simulink model "ACtoDC_WPT_current_DC"  (R2018a)
settings: Solver=FixedStepAuto  StartTime=0.0  StopTime=stopTime  FixedStep=sampleTime  RelTol=1e-3
InitFcn:
  | fs=150e3; %Hz
  | wo=2*pi*fs;
  | stopTime=0.1;
  | sampleTime=1e-8;
  | Lp=81e-6;
  | Ls=66e-6;
  | Cs=1/ (Ls*4*pi*pi*150e3*150e3);
  | Cp=1/ (Lp*4*pi*pi*150e3*150e3);
  | RLOAD=20
  | k=0.2;
  | M=sqrt(Lp*Ls)*k;
  | Cout=1e-6; %F
  | fs=150e3*sqrt(1+k^2); %Hz
values from neighbouring files (symbols this model uses):
  Rp = 0.3    [Calculation.m]
libraries: powerlib x37
settings Model: Creator=enes_  LastModifiedBy=enes_

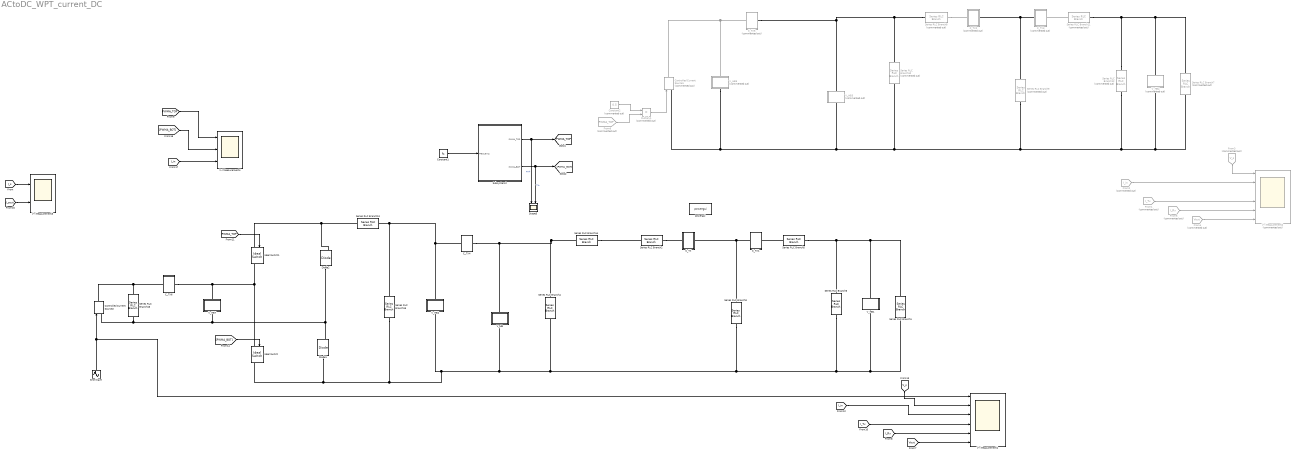
== system ACtoDC_WPT_current_DC ==
  C_TX : Subsystem
  C_TX1 : Subsystem
  C_TX2 : Subsystem  Commented=on
  C_TX3 : Subsystem  Commented=on
  C_TX4 : Subsystem
  C_TX5 : Subsystem  Commented=on
  C_TX6 : Subsystem
  Constant1 : Constant  Value=fs
  Constant2 : Constant  Commented=on  Value=0.5
  Controlled Current Source1 : powerlib/Electrical Sources/Controlled Current Source  Commented=on  Initialize=on  Source_Type=AC  Amplitude=0  Phase=0  Frequency=0  Measurements=None
  Controlled Current Source2 : powerlib/Electrical Sources/Controlled Current Source  Initialize=on  Source_Type=AC  Amplitude=0  Phase=0  Frequency=0  Measurements=None
  Diode1 : powerlib/Power Electronics/Diode  Ron=0.01  Lon=0  Vf=0.8  IC=0  UseSnubber=0  Rs=500  Cs=250e-9  Measurements=on
  Diode2 : powerlib/Power Electronics/Diode  Ron=0.01  Lon=0  Vf=0.8  IC=0  UseSnubber=0  Rs=500  Cs=250e-9  Measurements=on
  From1 : From  Commented=on  GotoTag=I_Tx  TagVisibility=global
  From2 : From  Commented=on  GotoTag=I_in  TagVisibility=global
  From3 : From  Commented=on  GotoTag=V_s  TagVisibility=global
  From4 : From  Commented=on  GotoTag=Vout  TagVisibility=global
  From5 : From  Commented=on  GotoTag=I_Rx  TagVisibility=global
  From6 : From  Commented=on  GotoTag=PWMA_TOP  TagVisibility=global
  Ideal Switch : powerlib/Power Electronics/Ideal Switch  Ron=0.01  Lon=0  IC=0  Rs=1e5  Cs=inf  Measurements=on
  Ideal Switch1 : powerlib/Power Electronics/Ideal Switch  Ron=0.01  Lon=0  IC=0  Rs=1e5  Cs=inf  Measurements=on
  Multiply1 : Product  Commented=on
  Scope3 : Scope  NumInputPorts=2
  Series RLC Branch1 : powerlib/Elements/Series RLC Branch  LConnTagsString=__new0  RConnTagsString=__new0  BranchType=R  Resistance=RLOAD*10  Inductance=Lp  SetiL0=off  InitialCurrent=0  Capacitance=Cp  Setx0=off  InitialVoltage=0  Measurements=None
  Series RLC Branch10 : powerlib/Elements/Series RLC Branch  Commented=on  LConnTagsString=__new0  RConnTagsString=__new0  BranchType=C  Resistance=Rp  Inductance=Lp  SetiL0=off  InitialCurrent=0  Capacitance=Cp  Setx0=off  InitialVoltage=0  Measurements=None
  Series RLC Branch11 : powerlib/Elements/Series RLC Branch  Commented=on  LConnTagsString=__new0  RConnTagsString=__new0  BranchType=L  Resistance=Rp  Inductance=Ls-M  SetiL0=off  InitialCurrent=0  Capacitance=Cp  Setx0=off  InitialVoltage=0  Measurements=None
  Series RLC Branch12 : powerlib/Elements/Series RLC Branch  Commented=on  LConnTagsString=__new0  RConnTagsString=__new0  BranchType=C  Resistance=Rp  Inductance=Lp  SetiL0=off  InitialCurrent=0  Capacitance=Cs  Setx0=off  InitialVoltage=0  Measurements=None
  Series RLC Branch13 : powerlib/Elements/Series RLC Branch  LConnTagsString=__new0  RConnTagsString=__new0  BranchType=R  Resistance=Rp  Inductance=Lp  SetiL0=off  InitialCurrent=0  Capacitance=0.01  Setx0=off  InitialVoltage=0  Measurements=None
  Series RLC Branch14 : powerlib/Elements/Series RLC Branch  LConnTagsString=__new0  RConnTagsString=__new0  BranchType=C  Resistance=Rp  Inductance=Lp  SetiL0=off  InitialCurrent=0  Capacitance=Cp*5  Setx0=off  InitialVoltage=0  Measurements=None
  Series RLC Branch15 : powerlib/Elements/Series RLC Branch  LConnTagsString=__new0  RConnTagsString=__new0  BranchType=R  Resistance=10e3  Inductance=Lp  SetiL0=off  InitialCurrent=0  Capacitance=0.01  Setx0=off  InitialVoltage=0  Measurements=None
  Series RLC Branch16 : powerlib/Elements/Series RLC Branch  LConnTagsString=__new0  RConnTagsString=__new0  BranchType=R  Resistance=10e3  Inductance=Lp  SetiL0=off  InitialCurrent=0  Capacitance=0.01  Setx0=off  InitialVoltage=0  Measurements=None
  Series RLC Branch2 : powerlib/Elements/Series RLC Branch  LConnTagsString=__new0  RConnTagsString=__new0  BranchType=L  Resistance=Rp  Inductance=Lp-M  SetiL0=off  InitialCurrent=0  Capacitance=Cp  Setx0=off  InitialVoltage=0  Measurements=None
  Series RLC Branch3 : powerlib/Elements/Series RLC Branch  LConnTagsString=__new0  RConnTagsString=__new0  BranchType=L  Resistance=Rp  Inductance=M  SetiL0=off  InitialCurrent=0  Capacitance=Cp  Setx0=off  InitialVoltage=0  Measurements=None
  Series RLC Branch4 : powerlib/Elements/Series RLC Branch  LConnTagsString=__new0  RConnTagsString=__new0  BranchType=C  Resistance=Rp  Inductance=Lp  SetiL0=off  InitialCurrent=0  Capacitance=Cp/5  Setx0=off  InitialVoltage=0  Measurements=None
  Series RLC Branch5 : powerlib/Elements/Series RLC Branch  LConnTagsString=__new0  RConnTagsString=__new0  BranchType=L  Resistance=Rp  Inductance=Ls-M  SetiL0=off  InitialCurrent=0  Capacitance=Cp  Setx0=off  InitialVoltage=0  Measurements=None
  Series RLC Branch6 : powerlib/Elements/Series RLC Branch  LConnTagsString=__new0  RConnTagsString=__new0  BranchType=C  Resistance=Rp  Inductance=Lp  SetiL0=off  InitialCurrent=0  Capacitance=Cs  Setx0=off  InitialVoltage=0  Measurements=None
  Series RLC Branch7 : powerlib/Elements/Series RLC Branch  Commented=on  LConnTagsString=__new0  RConnTagsString=__new0  BranchType=R  Resistance=RLOAD*10  Inductance=Lp  SetiL0=off  InitialCurrent=0  Capacitance=Cp  Setx0=off  InitialVoltage=0  Measurements=None
  Series RLC Branch8 : powerlib/Elements/Series RLC Branch  Commented=on  LConnTagsString=__new0  RConnTagsString=__new0  BranchType=L  Resistance=Rp  Inductance=Lp-M  SetiL0=off  InitialCurrent=0  Capacitance=Cp  Setx0=off  InitialVoltage=0  Measurements=None
  Series RLC Branch9 : powerlib/Elements/Series RLC Branch  Commented=on  LConnTagsString=__new0  RConnTagsString=__new0  BranchType=L  Resistance=Rp  Inductance=M  SetiL0=off  InitialCurrent=0  Capacitance=Cp  Setx0=off  InitialVoltage=0  Measurements=None
  Sine Wave : Sin  Frequency=2*pi*50  SampleTime=0
  Subsystem2 : Subsystem
  V-I Measurement1 : Scope  NumInputPorts=6
  V-I Measurement2 : Scope  Commented=on  NumInputPorts=6
  V-I Measurement3 : Scope  NumInputPorts=2
  V-I Measurement4 : Scope  NumInputPorts=3
  V_HB : Subsystem
  V_HB1 : Subsystem
  V_HB2 : Subsystem
  V_HB3 : Subsystem  Commented=on
  V_HB4 : Subsystem  Commented=on
  V_HB5 : Subsystem  Commented=on
  V_HB7 : Subsystem
  powergui : powerlib/powergui  Priority=1  SimulationMode=Discrete  SampleTime=sampleTime  frequency=60  Iterations=50  frequencyindice=0  Pbase=100e6  ErrMax=1e-4  UnitsV=kV  UnitsW=MW  buscounter=0  FunctionMessages=off  echomessages=off  EnableUseOfTLC=off  CurrentSourceSwitches=off  DisableSnubberDevices=off  DisableRonSwitches=off  DisableVfSwitches=off  DisplayEquations=off  SolverType=Tustin/Backward Euler (TBE)  Interpol=off  ExternalGateDelay=off  methode=off  Ts=100  x0status=blocks  SPID=off  SwTol=0  HookPort=off  RestoreLinks=warning  ResistiveCurrentMeasurement=off  Frange=[0:2:500]  Ylog=off  Xlog=on  ShowGrid=off  save=off  variable=ZData  structure=ScopeData2  ZoomFFT=off  StartTime=0.0  cycles=4  DisplayStyle=2  fundamental=100  FreqAxis=off  MaxFrequency=600e3  frequencyindicesteady=1  RmsSteady=1  display=off
  tag scope: PWMA_TOP=global
  wires:
  Subsystem2/2(PWMA_BOT) -> Scope3/2, [PWMA_BOT]  "TA-"
  Constant1/1 -> Subsystem2/1(Frequency)
  Subsystem2/1(PWMA_TOP) -> [PWMA_TOP], Scope3/1  "TA+"
  [Vout] -> V-I Measurement1/6
  [I_Rx] -> V-I Measurement1/5
  [I_Tx] -> V-I Measurement1/4
  From1/1 -> V-I Measurement2/4
  From3/1 -> V-I Measurement2/1
  From5/1 -> V-I Measurement2/5
  From4/1 -> V-I Measurement2/6
  Constant2/1 -> Multiply1/1
  From2/1 -> V-I Measurement2/2
  From6/1 -> Multiply1/2
  Multiply1/1 -> Controlled Current Source1/1
  [PWMA_BOT] -> Ideal Switch/1
  [PWMA_TOP] -> Ideal Switch1/1
  [I_s] -> V-I Measurement3/1
  [V_sout] -> V-I Measurement3/2
  [I_in] -> V-I Measurement1/3
  [V_s] -> V-I Measurement1/2
  [PWMA_TOP] -> V-I Measurement4/1
  [PWMA_BOT] -> V-I Measurement4/2
  [I_in] -> V-I Measurement4/3
  Sine Wave/1 -> V-I Measurement1/1, Controlled Current Source2/1
  connections:
  Diode1/LConn1 -- Ideal Switch/RConn1 -- Series RLC Branch15/LConn1 -- Series RLC Branch6/RConn1 -- V_HB1/LConn1 -- Series RLC Branch1/LConn1 -- Series RLC Branch3/RConn1 -- Series RLC Branch4/RConn1 -- V_HB/LConn1 -- V_HB2/LConn1
  Series RLC Branch5/LConn1 -- C_TX1/RConn1
  Series RLC Branch2/RConn1 -- C_TX/LConn1
  Series RLC Branch3/LConn1 -- C_TX1/LConn1 -- C_TX/RConn1
  Series RLC Branch5/RConn1 -- V_HB1/RConn1 -- Series RLC Branch1/RConn1 -- Series RLC Branch6/LConn1
  Series RLC Branch8/LConn1 -- Series RLC Branch10/LConn1 -- V_HB3/RConn1 -- C_TX5/RConn1
  Series RLC Branch7/LConn1 -- Controlled Current Source1/LConn1 -- V_HB5/LConn1 -- V_HB3/LConn1 -- Series RLC Branch10/RConn1 -- Series RLC Branch9/RConn1 -- Series RLC Branch12/RConn1 -- V_HB4/LConn1
  Series RLC Branch12/LConn1 -- Series RLC Branch11/RConn1 -- V_HB4/RConn1 -- Series RLC Branch7/RConn1
  C_TX2/RConn1 -- Series RLC Branch9/LConn1 -- C_TX3/LConn1
  C_TX5/LConn1 -- Controlled Current Source1/RConn1 -- V_HB5/RConn1
  Series RLC Branch8/RConn1 -- C_TX2/LConn1
  Series RLC Branch11/LConn1 -- C_TX3/RConn1
  Controlled Current Source2/RConn1 -- Series RLC Branch16/RConn1 -- C_TX6/LConn1
  V_HB7/LConn1 -- Diode2/LConn1 -- Diode1/RConn1 -- Series RLC Branch16/LConn1 -- Controlled Current Source2/LConn1
  C_TX4/LConn1 -- Series RLC Branch13/LConn1 -- Series RLC Branch15/RConn1 -- V_HB2/RConn1
  V_HB7/RConn1 -- Ideal Switch1/RConn1 -- Ideal Switch/LConn1 -- C_TX6/RConn1
  V_HB/RConn1 -- Series RLC Branch14/RConn1 -- Series RLC Branch4/LConn1 -- C_TX4/RConn1
  Ideal Switch1/LConn1 -- Diode2/RConn1 -- Series RLC Branch13/RConn1
  Series RLC Branch14/LConn1 -- Series RLC Branch2/LConn1

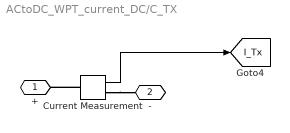
== system ACtoDC_WPT_current_DC/C_TX ==
  Current Measurement : powerlib/Measurements/Current Measurement  PhasorSimulation=off  OutputType=Complex  PSBequivalent=0
  + : PMIOPort  Side=Left
  - : PMIOPort  Port=2  Side=Right
  tag scope: I_Tx=global
  wires:
  Current Measurement/1 -> [I_Tx]
  connections:
  Current Measurement/RConn1 -- -/RConn1
  Current Measurement/LConn1 -- +/RConn1

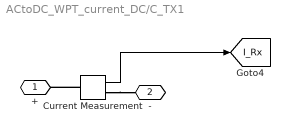
== system ACtoDC_WPT_current_DC/C_TX1 ==
  Current Measurement : powerlib/Measurements/Current Measurement  PhasorSimulation=off  OutputType=Complex  PSBequivalent=0
  + : PMIOPort  Side=Left
  - : PMIOPort  Port=2  Side=Right
  tag scope: I_Rx=global
  wires:
  Current Measurement/1 -> [I_Rx]
  connections:
  Current Measurement/RConn1 -- -/RConn1
  Current Measurement/LConn1 -- +/RConn1

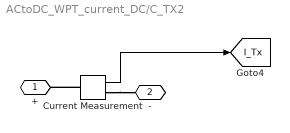
== system ACtoDC_WPT_current_DC/C_TX2 ==
  Current Measurement : powerlib/Measurements/Current Measurement  PhasorSimulation=off  OutputType=Complex  PSBequivalent=0
  + : PMIOPort  Side=Left
  - : PMIOPort  Port=2  Side=Right
  tag scope: I_Tx=global
  wires:
  Current Measurement/1 -> [I_Tx]
  connections:
  Current Measurement/RConn1 -- -/RConn1
  Current Measurement/LConn1 -- +/RConn1

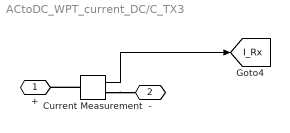
== system ACtoDC_WPT_current_DC/C_TX3 ==
  Current Measurement : powerlib/Measurements/Current Measurement  PhasorSimulation=off  OutputType=Complex  PSBequivalent=0
  + : PMIOPort  Side=Left
  - : PMIOPort  Port=2  Side=Right
  tag scope: I_Rx=global
  wires:
  Current Measurement/1 -> [I_Rx]
  connections:
  Current Measurement/RConn1 -- -/RConn1
  Current Measurement/LConn1 -- +/RConn1

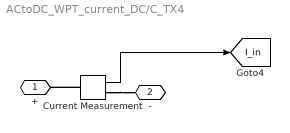
== system ACtoDC_WPT_current_DC/C_TX4 ==
  Current Measurement : powerlib/Measurements/Current Measurement  PhasorSimulation=off  OutputType=Complex  PSBequivalent=0
  + : PMIOPort  Side=Left
  - : PMIOPort  Port=2  Side=Right
  tag scope: I_in=global
  wires:
  Current Measurement/1 -> [I_in]
  connections:
  Current Measurement/RConn1 -- -/RConn1
  Current Measurement/LConn1 -- +/RConn1

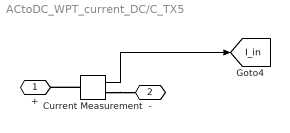
== system ACtoDC_WPT_current_DC/C_TX5 ==
  Current Measurement : powerlib/Measurements/Current Measurement  PhasorSimulation=off  OutputType=Complex  PSBequivalent=0
  + : PMIOPort  Side=Left
  - : PMIOPort  Port=2  Side=Right
  tag scope: I_in=global
  wires:
  Current Measurement/1 -> [I_in]
  connections:
  Current Measurement/RConn1 -- -/RConn1
  Current Measurement/LConn1 -- +/RConn1

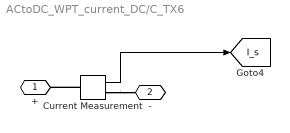
== system ACtoDC_WPT_current_DC/C_TX6 ==
  Current Measurement : powerlib/Measurements/Current Measurement  PhasorSimulation=off  OutputType=Complex  PSBequivalent=0
  + : PMIOPort  Side=Left
  - : PMIOPort  Port=2  Side=Right
  tag scope: I_s=global
  wires:
  Current Measurement/1 -> [I_s]
  connections:
  Current Measurement/RConn1 -- -/RConn1
  Current Measurement/LConn1 -- +/RConn1

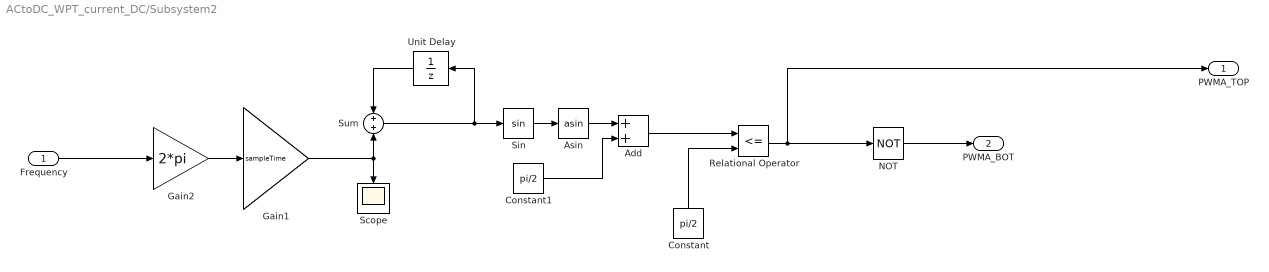
== system ACtoDC_WPT_current_DC/Subsystem2 ==
  Frequency : Inport
  Add : Sum
  Asin : Trigonometry  Operator=asin
  Constant : Constant  Value=pi/2
  Constant1 : Constant  Value=pi/2
  Gain1 : Gain  Gain=sampleTime
  Gain2 : Gain  Gain=2*pi
  NOT : Logic  Operator=NOT  IconShape=distinctive  AllPortsSameDT=off  OutDataTypeStr=boolean
  Relational Operator : RelationalOperator  Operator=<=  OutDataTypeStr=boolean  RndMeth=Simplest
  Scope : Scope
  Sin : Trigonometry
  Sum : Sum
  Unit Delay : UnitDelay  SampleTime=-1
  PWMA_TOP : Outport
  PWMA_BOT : Outport  Port=2
  wires:
  Gain1/1 -> Sum/2, Scope/1
  Asin/1 -> Add/1
  Sum/1 -> Sin/1, Unit Delay/1
  Gain2/1 -> Gain1/1
  Unit Delay/1 -> Sum/1
  Relational Operator/1 -> PWMA_TOP/1, NOT/1
  Frequency/1 -> Gain2/1
  Add/1 -> Relational Operator/1
  Sin/1 -> Asin/1
  Constant1/1 -> Add/2
  Constant/1 -> Relational Operator/2
  NOT/1 -> PWMA_BOT/1

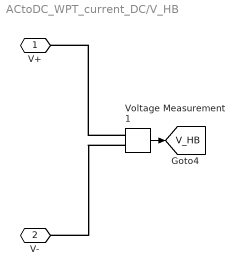
== system ACtoDC_WPT_current_DC/V_HB ==
  Voltage Measurement1 : powerlib/Measurements/Voltage Measurement  PhasorSimulation=off  OutputType=Complex  PSBequivalent=0
  V+ : PMIOPort  Side=Right
  V- : PMIOPort  Port=2  Side=Left
  tag scope: V_HB=global
  wires:
  Voltage Measurement1/1 -> [V_HB]
  connections:
  Voltage Measurement1/LConn1 -- V+/RConn1
  Voltage Measurement1/LConn2 -- V-/RConn1

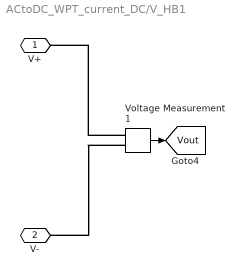
== system ACtoDC_WPT_current_DC/V_HB1 ==
  Voltage Measurement1 : powerlib/Measurements/Voltage Measurement  PhasorSimulation=off  OutputType=Complex  PSBequivalent=0
  V+ : PMIOPort  Side=Right
  V- : PMIOPort  Port=2  Side=Left
  tag scope: Vout=global
  wires:
  Voltage Measurement1/1 -> [Vout]
  connections:
  Voltage Measurement1/LConn1 -- V+/RConn1
  Voltage Measurement1/LConn2 -- V-/RConn1

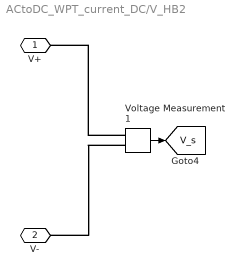
== system ACtoDC_WPT_current_DC/V_HB2 ==
  Voltage Measurement1 : powerlib/Measurements/Voltage Measurement  PhasorSimulation=off  OutputType=Complex  PSBequivalent=0
  V+ : PMIOPort  Side=Right
  V- : PMIOPort  Port=2  Side=Left
  tag scope: V_s=global
  wires:
  Voltage Measurement1/1 -> [V_s]
  connections:
  Voltage Measurement1/LConn1 -- V+/RConn1
  Voltage Measurement1/LConn2 -- V-/RConn1

== system ACtoDC_WPT_current_DC/V_HB3 ==
  Voltage Measurement1 : powerlib/Measurements/Voltage Measurement  PhasorSimulation=off  OutputType=Complex  PSBequivalent=0
  V+ : PMIOPort  Side=Right
  V- : PMIOPort  Port=2  Side=Left
  tag scope: V_HB=global
  wires:
  Voltage Measurement1/1 -> [V_HB]
  connections:
  Voltage Measurement1/LConn1 -- V+/RConn1
  Voltage Measurement1/LConn2 -- V-/RConn1

== system ACtoDC_WPT_current_DC/V_HB4 ==
  Voltage Measurement1 : powerlib/Measurements/Voltage Measurement  PhasorSimulation=off  OutputType=Complex  PSBequivalent=0
  V+ : PMIOPort  Side=Right
  V- : PMIOPort  Port=2  Side=Left
  tag scope: Vout=global
  wires:
  Voltage Measurement1/1 -> [Vout]
  connections:
  Voltage Measurement1/LConn1 -- V+/RConn1
  Voltage Measurement1/LConn2 -- V-/RConn1

== system ACtoDC_WPT_current_DC/V_HB5 ==
  Voltage Measurement1 : powerlib/Measurements/Voltage Measurement  PhasorSimulation=off  OutputType=Complex  PSBequivalent=0
  V+ : PMIOPort  Side=Right
  V- : PMIOPort  Port=2  Side=Left
  tag scope: V_s=global
  wires:
  Voltage Measurement1/1 -> [V_s]
  connections:
  Voltage Measurement1/LConn1 -- V+/RConn1
  Voltage Measurement1/LConn2 -- V-/RConn1

== system ACtoDC_WPT_current_DC/V_HB7 ==
  Voltage Measurement1 : powerlib/Measurements/Voltage Measurement  PhasorSimulation=off  OutputType=Complex  PSBequivalent=0
  V+ : PMIOPort  Side=Right
  V- : PMIOPort  Port=2  Side=Left
  tag scope: V_sout=global
  wires:
  Voltage Measurement1/1 -> [V_sout]
  connections:
  Voltage Measurement1/LConn1 -- V+/RConn1
  Voltage Measurement1/LConn2 -- V-/RConn1
